simulink library "engine_JetCatP70_lib"  (Simulink 7.2)
settings: Solver=ode45  SolverMode=SingleTasking  StartTime=0.0  StopTime=10.0  RelTol=1e-3
libraries: simulink x1
settings Model: Creator=amurch  LastModifiedBy=E183308

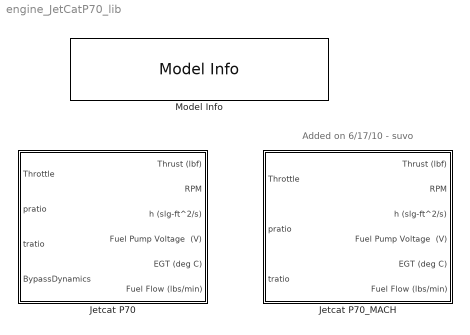
== system engine_JetCatP70_lib ==
  note: Added on 6/17/10 - suvo
  Jetcat P70 : Subsystem
      mask init:
      | % Curve fit parameters for Jetcat P70 Model
      | % Coeff_thrust   = [0.000028864242464  -0.001914835880159 0.105916926095459  -1.251646340183624 ];
      | Coeff_thrust   = [0.000014847593013,  0, 0, 0.412662356277121];
      | Coeff_throttle = [0.000033035538475  -0.008354385314499 1.191126728328792 31.518959847101669];
      | Coeff_fuelflow = [0.000046800927870  -0.000779344124807 0.122178501497750];
      | Coeff_tau      = [ -2.2400e-02   2.9948e+00];
      | Coeff_EGT      = [ 2E-5, -0.0036,0.2342,-8.0496,664.99]; %EGT model, deg C
      | Coeff_dynamics = [ -.074 7.1];
      | fuelpump_table = [0 0.576	0.625	0.6985	0.7845	0.8575	0.919	0.9805	1.0415	1.1025...
      |                     1.1515	1.262	1.287	1.373	1.52	1.618	1.74	1.887	1.973...
      |                     2.12	2.255	2.4385	2.647	2.7575	2.9905	3.162]; %volts, table of fuel pump voltages
      | fuelflow_table = [0,0.0794,0.0876,0.102,0.1149,0.1275,0.1379,0.1487,0.1586,0.1671,...
      |                     0.1775,0.1858,0.194,0.2038,0.2206,0.2405,0.2566,0.2746,0.2921,0.3102,...
      |                     0.3266,0.3445,0.3533,0.3611,0.3866,0.4083;]*2; %lbs/min,   FULL fuel flow rates corresponding to pump voltages (fuelpump_table)  
      | % Equvalent Shaft parameters for engine
      | shaft_dia = 0.75/12.0;       % diameter of rotating turbine in feet 
      | shaft_len = 6.25/12.0;       % length of rotating turbine in feet   
      | density   = 15.2;            % mass density of steel in slugs/ft^3 
      | 
      | 
      | A = [-1.336,-0.7314;1,0;];
      | B = [1;0];
      | C = [-0.1474   0.7314];
      | D = 0;
  Jetcat P70_MACH : Subsystem
      mask init: same as engine_JetCatP70_lib/Jetcat P70
  Model Info : simulink/Model-Wide Utilities/Model Info  SystemSampleTime=-1  InitialBlockCM=None  BlockCM=None  Frame=on  DisplayStringWithTags=|  HorizontalTextAlignment=Center  LeftAlignmentValue=0.5  SourceBlockDiagram=engine_JetCatP70_lib  TagMaxNumber=20
      | JetCat P70 Engine Library
      | 
      | Model Version: %<ModelVersion>
      | Last modifed by %<LastModifiedBy> on %<LastModificationDate>

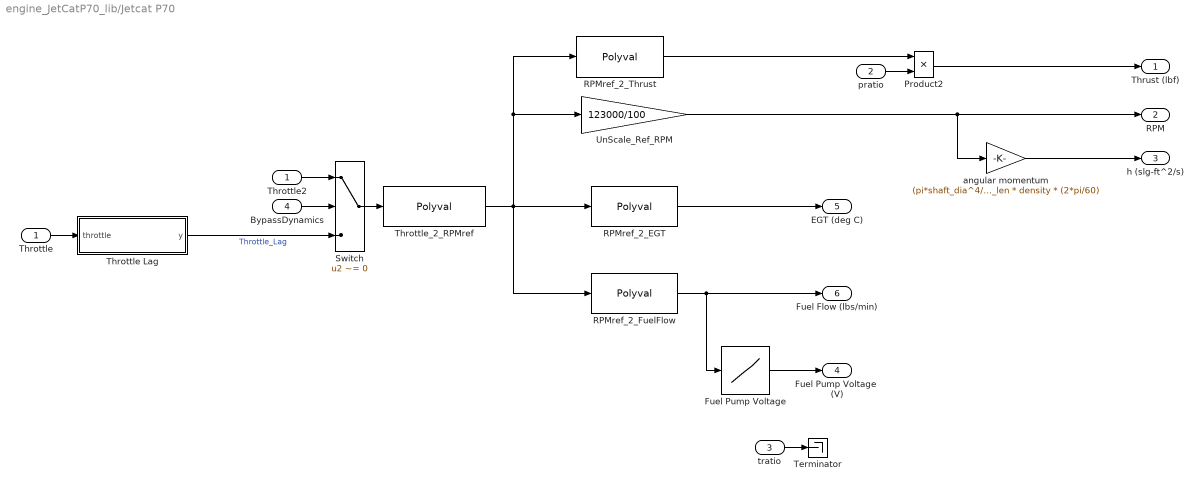
== system engine_JetCatP70_lib/Jetcat P70 ==
  Throttle : Inport  OutDataType=sfix(16)  OutScaling=2^0
  pratio : Inport  Port=2  OutDataType=sfix(16)  OutScaling=2^0
  tratio : Inport  Port=3  OutDataType=sfix(16)  OutScaling=2^0
  BypassDynamics : Inport  Port=4  OutDataType=sfix(16)  OutScaling=2^0
  Fuel Pump Voltage : Lookup  InputValues=fuelflow_table  Table=fuelpump_table  LookUpMeth=Interpolation-Use End Values  OutDataType=sfix(16)  OutScaling=2^0
  Product2 : Product  OutDataType=sfix(16)  OutScaling=2^0  RndMeth=Zero
  RPMref_2_EGT : Polyval  Coefs=Coeff_EGT
  RPMref_2_FuelFlow : Polyval  Coefs=Coeff_fuelflow
  RPMref_2_Thrust : Polyval  Coefs=Coeff_thrust
  Switch : Switch  Criteria=u2 ~= 0
  Terminator : Terminator
  Throttle Lag : Subsystem
  Throttle2 : InportShadow  Port=1  OutDataType=sfix(16)  OutScaling=2^0  LatchByCopyingInsideSignal=off
  Throttle_2_RPMref : Polyval  Coefs=Coeff_throttle
  UnScale_Ref_RPM : Gain  Gain=123000/100  ParameterDataType=sfix(16)  ParameterScaling=2^0  OutDataType=sfix(16)  OutScaling=2^0
  angular momentum : Gain  Gain=(pi*shaft_dia^4/32) * shaft_len * density * (2*pi/60)  ParameterDataType=sfix(16)  ParameterScaling=2^0  OutDataType=sfix(16)  OutScaling=2^0
  Thrust (lbf) : Outport  OutDataType=sfix(16)  OutScaling=2^0
  RPM : Outport  Port=2  OutDataType=sfix(16)  OutScaling=2^0
  h (slg-ft^2/s) : Outport  Port=3  OutDataType=sfix(16)  OutScaling=2^0
  Fuel Pump Voltage  (V) : Outport  Port=4  OutDataType=sfix(16)  OutScaling=2^0
  EGT (deg C) : Outport  Port=5  OutDataType=sfix(16)  OutScaling=2^0
  Fuel Flow (lbs/min) : Outport  Port=6  OutDataType=sfix(16)  OutScaling=2^0
  wires:
  RPMref_2_EGT/1 -> EGT (deg C)/1
  Fuel Pump Voltage/1 -> Fuel Pump Voltage  (V)/1
  pratio/1 -> Product2/2
  RPMref_2_FuelFlow/1 -> Fuel Pump Voltage/1, Fuel Flow (lbs/min)/1
  Product2/1 -> Thrust (lbf)/1
  RPMref_2_Thrust/1 -> Product2/1
  tratio/1 -> Terminator/1
  UnScale_Ref_RPM/1 -> RPM/1, angular momentum/1
  angular momentum/1 -> h (slg-ft^2/s)/1
  Throttle_2_RPMref/1 -> RPMref_2_EGT/1, UnScale_Ref_RPM/1, RPMref_2_Thrust/1, RPMref_2_FuelFlow/1
  Throttle/1 -> Throttle Lag/1(throttle)
  Switch/1 -> Throttle_2_RPMref/1
  Throttle Lag/1(y) -> Switch/3  "Throttle_Lag"
  BypassDynamics/1 -> Switch/2
  Throttle2/1 -> Switch/1

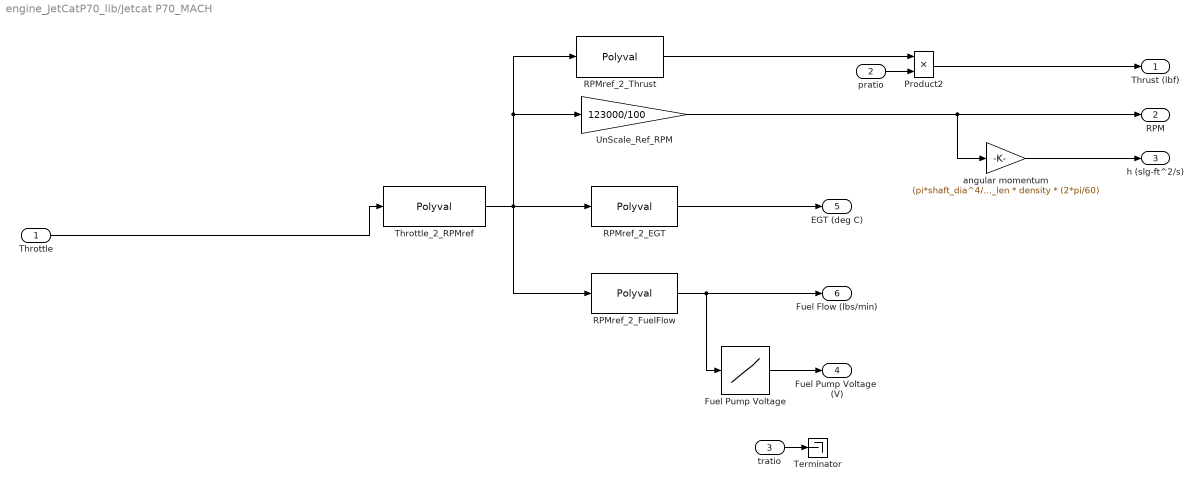
== system engine_JetCatP70_lib/Jetcat P70_MACH ==
  Throttle : Inport  OutDataType=sfix(16)  OutScaling=2^0
  pratio : Inport  Port=2  OutDataType=sfix(16)  OutScaling=2^0
  tratio : Inport  Port=3  OutDataType=sfix(16)  OutScaling=2^0
  Fuel Pump Voltage : Lookup  InputValues=fuelflow_table  Table=fuelpump_table  LookUpMeth=Interpolation-Use End Values  OutDataType=sfix(16)  OutScaling=2^0
  Product2 : Product  OutDataType=sfix(16)  OutScaling=2^0  RndMeth=Zero
  RPMref_2_EGT : Polyval  Coefs=Coeff_EGT
  RPMref_2_FuelFlow : Polyval  Coefs=Coeff_fuelflow
  RPMref_2_Thrust : Polyval  Coefs=Coeff_thrust
  Terminator : Terminator
  Throttle_2_RPMref : Polyval  Coefs=Coeff_throttle
  UnScale_Ref_RPM : Gain  Gain=123000/100  ParameterDataType=sfix(16)  ParameterScaling=2^0  OutDataType=sfix(16)  OutScaling=2^0
  angular momentum : Gain  Gain=(pi*shaft_dia^4/32) * shaft_len * density * (2*pi/60)  ParameterDataType=sfix(16)  ParameterScaling=2^0  OutDataType=sfix(16)  OutScaling=2^0
  Thrust (lbf) : Outport  OutDataType=sfix(16)  OutScaling=2^0
  RPM : Outport  Port=2  OutDataType=sfix(16)  OutScaling=2^0
  h (slg-ft^2/s) : Outport  Port=3  OutDataType=sfix(16)  OutScaling=2^0
  Fuel Pump Voltage  (V) : Outport  Port=4  OutDataType=sfix(16)  OutScaling=2^0
  EGT (deg C) : Outport  Port=5  OutDataType=sfix(16)  OutScaling=2^0
  Fuel Flow (lbs/min) : Outport  Port=6  OutDataType=sfix(16)  OutScaling=2^0
  wires:
  Throttle/1 -> Throttle_2_RPMref/1
  Throttle_2_RPMref/1 -> RPMref_2_FuelFlow/1, RPMref_2_Thrust/1, UnScale_Ref_RPM/1, RPMref_2_EGT/1
  angular momentum/1 -> h (slg-ft^2/s)/1
  UnScale_Ref_RPM/1 -> angular momentum/1, RPM/1
  tratio/1 -> Terminator/1
  RPMref_2_Thrust/1 -> Product2/1
  Product2/1 -> Thrust (lbf)/1
  RPMref_2_FuelFlow/1 -> Fuel Flow (lbs/min)/1, Fuel Pump Voltage/1
  pratio/1 -> Product2/2
  Fuel Pump Voltage/1 -> Fuel Pump Voltage  (V)/1
  RPMref_2_EGT/1 -> EGT (deg C)/1

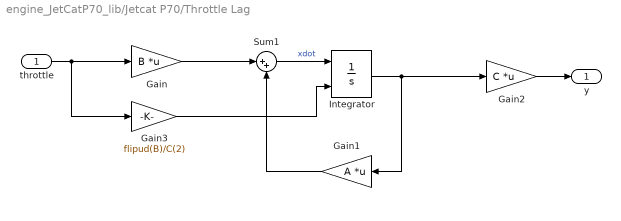
== system engine_JetCatP70_lib/Jetcat P70/Throttle Lag ==
  throttle : Inport  OutDataType=sfix(16)  OutScaling=2^0
  Gain : Gain  Gain=B  Multiplication=Matrix(K*u)  ParameterDataType=sfix(16)  ParameterScaling=2^0  OutDataType=sfix(16)  OutScaling=2^0
  Gain1 : Gain  Orientation=left  Gain=A  Multiplication=Matrix(K*u)  ParameterDataType=sfix(16)  ParameterScaling=2^0  OutDataType=sfix(16)  OutScaling=2^0
  Gain2 : Gain  Gain=C  Multiplication=Matrix(K*u)  ParameterDataType=sfix(16)  ParameterScaling=2^0  OutDataType=sfix(16)  OutScaling=2^0
  Gain3 : Gain  Gain=flipud(B)/C(2)  ParameterDataType=sfix(16)  ParameterScaling=2^0  OutDataType=sfix(16)  OutScaling=2^0
  Integrator : Integrator  InitialConditionSource=external
  Sum1 : Sum  Inputs=|++  OutDataType=sfix(16)  OutScaling=2^0
  y : Outport  OutDataType=sfix(16)  OutScaling=2^0
  wires:
  Sum1/1 -> Integrator/1  "xdot"
  Gain1/1 -> Sum1/2
  Integrator/1 -> Gain1/1, Gain2/1
  Gain/1 -> Sum1/1
  Gain2/1 -> y/1
  throttle/1 -> Gain/1, Gain3/1
  Gain3/1 -> Integrator/2
